simulink model "models_continuosAndDiscrit_stepInput"  (R2021a)
settings: Solver=ode1  StartTime=0.0  StopTime=10.0  FixedStep=integration_step_size  RelTol=1e-3
values from neighbouring files (symbols this model uses):
  Gq = c2d(Gs,Ts,'zoh')    [list1.m]
  Gs = tf(K,[tal 1],'InputDelay',theta)    [list1.m]
  Ts = 1    [list1.m]
settings Model: Creator=Fernando  LastModifiedBy=Fernando

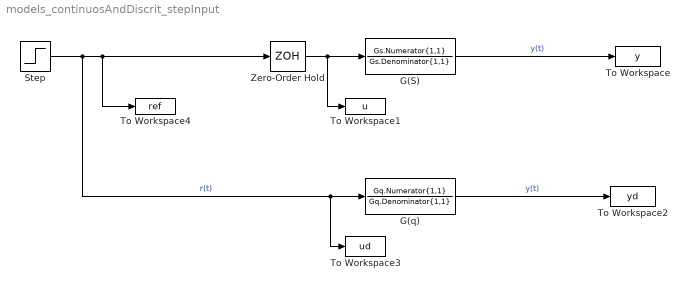
== system models_continuosAndDiscrit_stepInput ==
  G(S) : TransferFcn  Numerator=Gs.Numerator{1,1}  Denominator=Gs.Denominator{1,1}
  G(q) : DiscreteTransferFcn  Numerator=Gq.Numerator{1,1}  Denominator=Gq.Denominator{1,1}  SampleTime=Ts
  Step : Step  Time=0  After=0.1  SampleTime=0
  To Workspace : ToWorkspace  VariableName=y  SaveFormat=Timeseries  SampleTime=-1
      settings: Decimation=100
  To Workspace1 : ToWorkspace  VariableName=u  SaveFormat=Timeseries  SampleTime=-1
      settings: Decimation=100
  To Workspace2 : ToWorkspace  VariableName=yd  SaveFormat=Timeseries  SampleTime=-1
  To Workspace3 : ToWorkspace  VariableName=ud  SaveFormat=Timeseries  SampleTime=Ts
  To Workspace4 : ToWorkspace  VariableName=ref  SaveFormat=Timeseries  SampleTime=-1
      settings: Decimation=100
  Zero-Order Hold : ZeroOrderHold  SampleTime=-1
  wires:
  Step/1 -> To Workspace3/1, G(q)/1, Zero-Order Hold/1, To Workspace4/1  "r(t)"
  G(S)/1 -> To Workspace/1  "y(t)"
  G(q)/1 -> To Workspace2/1  "y(t)"
  Zero-Order Hold/1 -> To Workspace1/1, G(S)/1
